simulink model "mdl"  (R2020a)
settings: Solver=VariableStepAuto  StartTime=0.0  StopTime=100  RelTol=1e-3
values from neighbouring files (symbols this model uses):
  C = 2267000    [startup.m]
  H_l = 1050    [startup.m]
  n0_S = 1322    [startup.m]
  P_cp = 1924000    [startup.m]
libraries: simulink x1
settings Model: Creator=wenap  LastModifiedBy=jorge
settings DebuggingCC: SFMachineParentedDataDiag=error

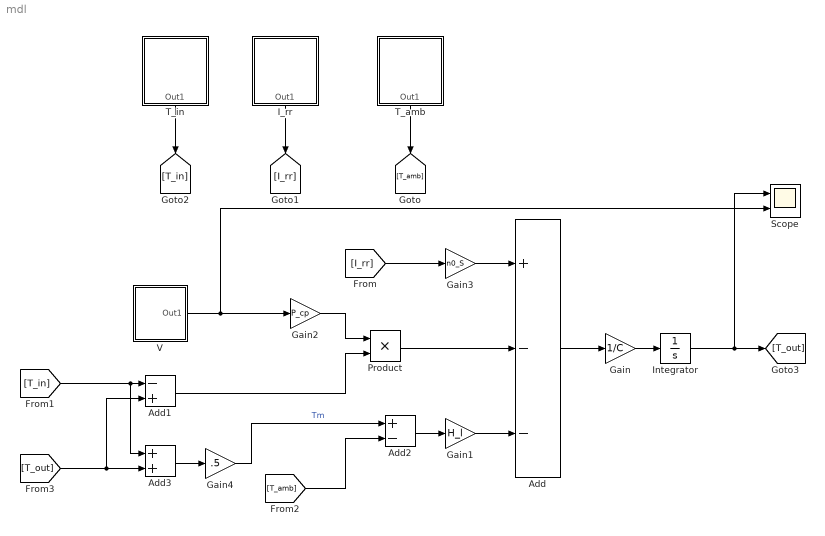
== system mdl ==
  Add : Sum  Inputs=+--
  Add1 : Sum  Inputs=-+
  Add2 : Sum  Inputs=+-
  Add3 : Sum
  Gain : Gain  Gain=1/C
  Gain1 : Gain  Gain=H_l
  Gain2 : Gain  Gain=P_cp
  Gain3 : Gain  Gain=n0_S
  Gain4 : Gain  Gain=.5
  I_rr : Subsystem
  Integrator : Integrator
  Product : Product
  Scope : Scope  NumInputPorts=2
  T_amb : Subsystem
  T_in : Subsystem
  V : Subsystem
  wires:
  Gain3/1 -> Add/1
  Add1/1 -> Product/2
  Gain2/1 -> Product/1
  Product/1 -> Add/2
  Add/1 -> Gain/1
  Gain1/1 -> Add/3
  Add2/1 -> Gain1/1
  V/1(Out1) -> Scope/2, Gain2/1
  Add3/1 -> Gain4/1
  Gain4/1 -> Add2/1  "Tm"
  T_in/1(Out1) -> [T_in]
  I_rr/1(Out1) -> [I_rr]
  T_amb/1(Out1) -> [T_amb]
  [I_rr] -> Gain3/1
  [T_in] -> Add3/1, Add1/1
  [T_amb] -> Add2/2
  Integrator/1 -> Scope/1, [T_out]
  [T_out] -> Add3/2, Add1/2
  Gain/1 -> Integrator/1

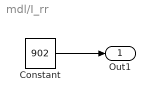
== system mdl/I_rr ==
  Constant : Constant  Value=902
  Out1 : Outport
  wires:
  Constant/1 -> Out1/1

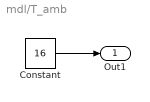
== system mdl/T_amb ==
  Constant : Constant  Value=16
  Out1 : Outport
  wires:
  Constant/1 -> Out1/1

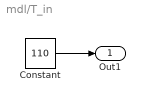
== system mdl/T_in ==
  Constant : Constant  Value=110
  Out1 : Outport
  wires:
  Constant/1 -> Out1/1

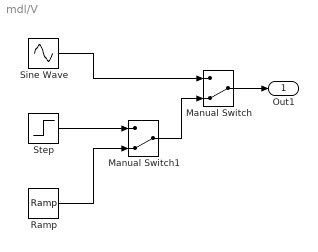
== system mdl/V ==
  Manual Switch : ManualSwitch  CurrentSetting=0
  Manual Switch1 : ManualSwitch  CurrentSetting=0
  Ramp : simulink/Sources/Ramp  slope=0.1  start=10  InitialOutput=0
  Sine Wave : Sin  Bias=1  SampleTime=0
  Step : Step  Time=10  After=7  SampleTime=0
  Out1 : Outport
  wires:
  Sine Wave/1 -> Manual Switch/1
  Step/1 -> Manual Switch1/1
  Manual Switch/1 -> Out1/1
  Ramp/1 -> Manual Switch1/2
  Manual Switch1/1 -> Manual Switch/2
